simulink library "lib_ares"  (R2020a)
settings: Solver=VariableStepAuto  StartTime=0.0  StopTime=10.0  RelTol=1e-3
undefined symbols (not defined in the file or in its folder): DiscIntNeverNeededParam
libraries: simulink x9, $bdroot x6
(part 2 of 2)

== system lib_ares/baro_alt_to_Ps ==
  note: Static Pressure (atmospheres) as a function of Baro Alt (ft)
      | (valid for Alt < 36089)
      | this is /delta
  baro_alt_ft : Inport
  baro_alt_ft_to_Ps_atm : Fcn  Expr=(1.0-(u*(0.00356616/518.67)))^5.2561
  Ps_atm : Outport
  wires:
  baro_alt_ft/1 -> baro_alt_ft_to_Ps_atm/1
  baro_alt_ft_to_Ps_atm/1 -> Ps_atm/1

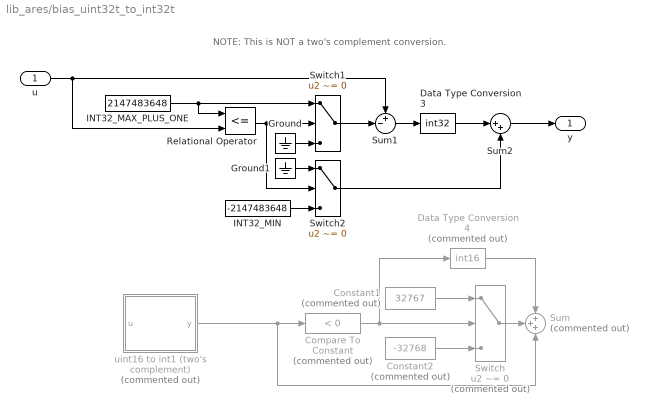
== system lib_ares/bias_uint32t_to_int32t ==
  note: NOTE: This is NOT a two's complement conversion.
  u : Inport  OutDataTypeStr=uint32
  Compare To Constant : simulink/Logic and Bit Operations/Compare To Constant  Commented=on  relop=<  const=0  OutDataTypeStr=boolean
  Constant1 : Constant  Commented=on  Value=32767  VectorParams1D=off  OutDataTypeStr=int16  SampleTime=1e-6
  Constant2 : Constant  Commented=on  Value=-32768  OutDataTypeStr=int16  SampleTime=1e-6
  Data Type Conversion3 : DataTypeConversion  OutDataTypeStr=int32  SaturateOnIntegerOverflow=on
  Data Type Conversion4 : DataTypeConversion  Commented=on  OutDataTypeStr=int16  SaturateOnIntegerOverflow=on
  Ground : Ground
  Ground1 : Ground
  INT32_MAX_PLUS_ONE : Constant  Value=2147483648  OutDataTypeStr=uint32
  INT32_MIN : Constant  Value=-2147483648  OutDataTypeStr=int32
  Relational Operator : RelationalOperator  Operator=<=  OutDataTypeStr=boolean  RndMeth=Simplest
  Sum : Sum  Commented=on  Inputs=+++
  Sum1 : Sum  Inputs=+-|
  Sum2 : Sum  Inputs=|++
  Switch : Switch  Commented=on  Criteria=u2 ~= 0
  Switch1 : Switch  Criteria=u2 ~= 0
  Switch2 : Switch  Criteria=u2 ~= 0
  uint16 to int1 (two's complement) : Subsystem  Commented=on
  y : Outport  OutDataTypeStr=int32
  wires:
  uint16 to int1 (two's complement)/1(y) -> Compare To Constant/1, Sum/3
  Data Type Conversion4/1 -> Sum/1
  Compare To Constant/1 -> Switch/2, Data Type Conversion4/1
  Constant2/1 -> Switch/3
  Constant1/1 -> Switch/1
  Switch/1 -> Sum/2
  ? -> uint16 to int1 (two's complement)/1(u)
  Sum2/1 -> y/1
  Switch1/1 -> Sum1/2
  INT32_MIN/1 -> Switch2/3
  INT32_MAX_PLUS_ONE/1 -> Relational Operator/1, Switch1/1
  Sum1/1 -> Data Type Conversion3/1
  Relational Operator/1 -> Switch1/2, Switch2/2
  Data Type Conversion3/1 -> Sum2/1
  Switch2/1 -> Sum2/2
  Ground/1 -> Switch1/3
  Ground1/1 -> Switch2/1
  u/1 -> Sum1/1, Relational Operator/2

== system lib_ares/cas_to_mach ==
  note: Mach number as a function of
      | calibrated airspeed (ft/s)
      |
      | NASA Reference Publication 1046, Pg.15 Speed of Sound
  cas_fps : Inport
  Divide : Product  Inputs=*/
  "Speed of Sound, fps, Sea Level Standard" : Constant  Value=1116.450  OutDataTypeStr=Inherit: Inherit via back propagation
  mach : Outport
  wires:
  "Speed of Sound, fps, Sea Level Standard"/1 -> Divide/2
  cas_fps/1 -> Divide/1
  Divide/1 -> mach/1

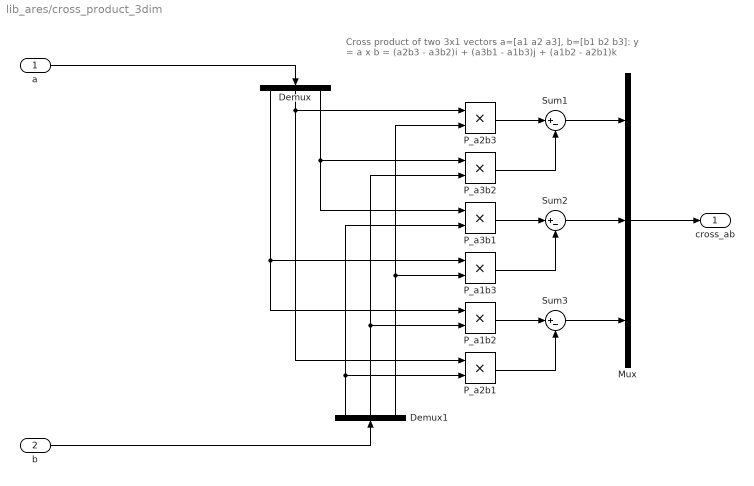
== system lib_ares/cross_product_3dim ==
  note: Cross product of two 3x1 vectors a=[a1 a2 a3], b=[b1 b2 b3]:
      | y = a x b = (a2b3 - a3b2)i + (a3b1 - a1b3)j + (a1b2 - a2b1)k
  a : Inport
  b : Inport  Port=2
  Demux : Demux  Outputs=3
  Demux1 : Demux  Outputs=3
  Mux : Mux  Inputs=3
  P_a1b2 : Product
  P_a1b3 : Product
  P_a2b1 : Product
  P_a2b3 : Product
  P_a3b1 : Product
  P_a3b2 : Product
  Sum1 : Sum  Inputs=|+-
  Sum2 : Sum  Inputs=|+-
  Sum3 : Sum  Inputs=|+-
  cross_ab : Outport
  wires:
  Demux/1 -> P_a1b3/1, P_a1b2/1
  Demux1/1 -> P_a3b1/2, P_a2b1/2
  Demux/2 -> P_a2b1/1, P_a2b3/1
  Demux/3 -> P_a3b1/1, P_a3b2/1
  P_a1b3/1 -> Sum2/2
  P_a2b1/1 -> Sum3/2
  P_a1b2/1 -> Sum3/1
  Demux1/3 -> P_a2b3/2, P_a1b3/2
  Demux1/2 -> P_a3b2/2, P_a1b2/2
  P_a3b2/1 -> Sum1/2
  P_a3b1/1 -> Sum2/1
  P_a2b3/1 -> Sum1/1
  Sum2/1 -> Mux/2
  Sum1/1 -> Mux/1
  Sum3/1 -> Mux/3
  b/1 -> Demux1/1
  a/1 -> Demux/1
  Mux/1 -> cross_ab/1

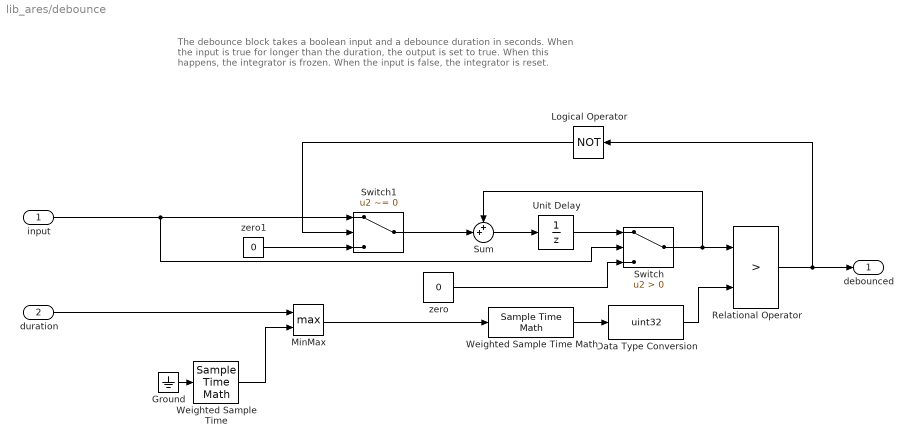
== system lib_ares/debounce ==
  note: The debounce block takes a boolean input and a debounce duration in seconds.
      |
      | When the input is true for longer than the duration, the output is set to true. When
      | this happens, the integrator is frozen. When the input is false, the integrator is
      | reset.
  input : Inport  OutDataTypeStr=boolean
  duration : Inport  Port=2
  Data Type Conversion : DataTypeConversion  OutDataTypeStr=uint32
  Ground : Ground
  Logical Operator : Logic  Operator=NOT  AllPortsSameDT=off  OutDataTypeStr=boolean
  MinMax : MinMax  Function=max  Inputs=2
  Relational Operator : RelationalOperator  Operator=>  OutDataTypeStr=boolean  RndMeth=Simplest
  Sum : Sum  Inputs=++|
  Switch : Switch  Criteria=u2 > Threshold
  Switch1 : Switch  Criteria=u2 ~= 0
  Unit Delay : UnitDelay  SampleTime=-1  HasFrameUpgradeWarning=on
  Weighted Sample Time : SampleTimeMath  TsampMathOp=Ts Only
  Weighted Sample Time Math : SampleTimeMath  TsampMathOp=/
  zero : Constant  Value=0  OutDataTypeStr=uint32
  zero1 : Constant  Value=0  OutDataTypeStr=uint32
  debounced : Outport  VectorParamsAs1DForOutWhenUnconnected=off
  wires:
  zero1/1 -> Switch1/3
  Logical Operator/1 -> Switch1/2
  Switch1/1 -> Sum/2
  input/1 -> Switch1/1, Switch/2
  Switch/1 -> Relational Operator/1, Sum/1
  Unit Delay/1 -> Switch/1
  Weighted Sample Time Math/1 -> Data Type Conversion/1
  zero/1 -> Switch/3
  Sum/1 -> Unit Delay/1
  duration/1 -> MinMax/1
  Relational Operator/1 -> debounced/1, Logical Operator/1
  MinMax/1 -> Weighted Sample Time Math/1
  Weighted Sample Time/1 -> MinMax/2
  Ground/1 -> Weighted Sample Time/1
  Data Type Conversion/1 -> Relational Operator/2

== system lib_ares/fta_handler_non_persistent ==
  input : Inport
  id : Inport  Port=2
  enable : Inport  Port=3
  Data Type Duplicate : DataTypeDuplicate
  Logical Operator3 : Logic  AllPortsSameDT=off  OutDataTypeStr=boolean
  Relational Operator2 : RelationalOperator  Operator===  OutDataTypeStr=boolean  RndMeth=Simplest
  Switch3 : Switch  Criteria=u2 ~= 0
  default_value_IC : Constant  Value=default_value  OutDataTypeStr=Inherit: Inherit via back propagation
  id_int32 : Constant  Value=id  OutDataTypeStr=int32
  output : Outport
  wires:
  id_int32/1 -> Relational Operator2/1
  input/1 -> Data Type Duplicate/1, Switch3/1  "new_value"
  Relational Operator2/1 -> Logical Operator3/1
  Switch3/1 -> output/1
  id/1 -> Relational Operator2/2
  enable/1 -> Logical Operator3/2
  default_value_IC/1 -> Data Type Duplicate/2, Switch3/3  "default_value"
  Logical Operator3/1 -> Switch3/2

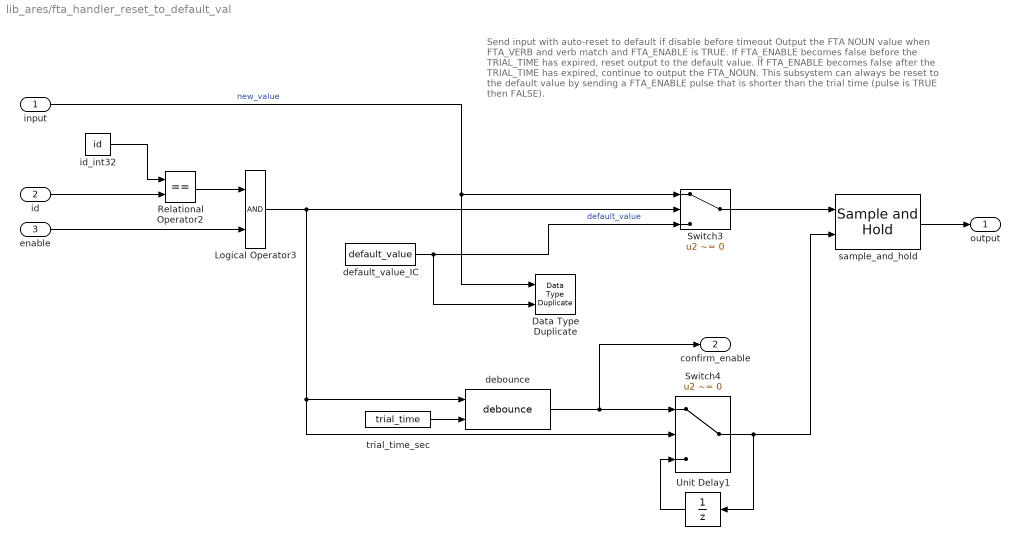
== system lib_ares/fta_handler_reset_to_default_val ==
  note: Send input with auto-reset to default if disable before timeout
      |
      | Output the FTA NOUN value when FTA_VERB and verb match and FTA_ENABLE is TRUE.
      | If FTA_ENABLE becomes false before the TRIAL_TIME has expired, reset output to the
      | default value. If FTA_ENABLE becomes false after the TRIAL_TIME has expired, continue
      | to output the FTA_NOUN.
      |
      | This subsystem can always be reset to the default value by sending a FTA_ENABLE pulse
      | that is shorter than the trial time (pulse is TRUE then FALSE).
  input : Inport
  id : Inport  Port=2
  enable : Inport  Port=3
  Data Type Duplicate : DataTypeDuplicate
  Logical Operator3 : Logic  AllPortsSameDT=off  OutDataTypeStr=boolean
  Relational Operator2 : RelationalOperator  Operator===  OutDataTypeStr=boolean  RndMeth=Simplest
  Switch3 : Switch  Criteria=u2 ~= 0
  Switch4 : Switch  Criteria=u2 ~= 0
  Unit Delay1 : UnitDelay  SampleTime=-1  HasFrameUpgradeWarning=on
  debounce : $bdroot/debounce  SystemSampleTime=-1  Latency=0  AutoFrameSizeCalculation=off
  default_value_IC : Constant  Value=default_value  OutDataTypeStr=Inherit: Inherit via back propagation
  id_int32 : Constant  Value=id  OutDataTypeStr=int32
  sample_and_hold : $bdroot/Sample and Hold  SystemSampleTime=-1  Latency=0  AutoFrameSizeCalculation=off
  trial_time_sec : Constant  Value=trial_time  OutDataTypeStr=Inherit: Inherit via back propagation
  output : Outport
  confirm_enable : Outport  Port=2
  wires:
  Logical Operator3/1 -> debounce/1, Switch4/2, Switch3/2
  debounce/1 -> confirm_enable/1, Switch4/1
  Unit Delay1/1 -> Switch4/3
  default_value_IC/1 -> Data Type Duplicate/2, Switch3/3  "default_value"
  enable/1 -> Logical Operator3/2
  id/1 -> Relational Operator2/2
  sample_and_hold/1 -> output/1
  Relational Operator2/1 -> Logical Operator3/1
  trial_time_sec/1 -> debounce/2
  Switch3/1 -> sample_and_hold/1
  input/1 -> Data Type Duplicate/1, Switch3/1  "new_value"
  id_int32/1 -> Relational Operator2/1
  Switch4/1 -> sample_and_hold/2, Unit Delay1/1

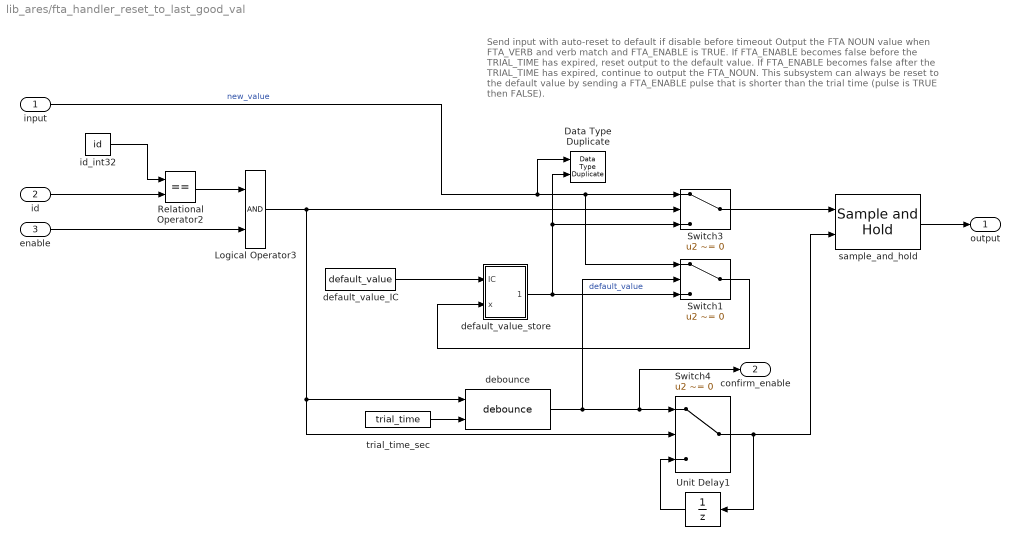
== system lib_ares/fta_handler_reset_to_last_good_val ==
  note: Send input with auto-reset to default if disable before timeout
      |
      | Output the FTA NOUN value when FTA_VERB and verb match and FTA_ENABLE is TRUE.
      | If FTA_ENABLE becomes false before the TRIAL_TIME has expired, reset output to the
      | default value. If FTA_ENABLE becomes false after the TRIAL_TIME has expired, continue
      | to output the FTA_NOUN.
      |
      | This subsystem can always be reset to the default value by sending a FTA_ENABLE pulse
      | that is shorter than the trial time (pulse is TRUE then FALSE).
  input : Inport
  id : Inport  Port=2
  enable : Inport  Port=3
  Data Type Duplicate : DataTypeDuplicate
  Logical Operator3 : Logic  AllPortsSameDT=off  OutDataTypeStr=boolean
  Relational Operator2 : RelationalOperator  Operator===  OutDataTypeStr=boolean  RndMeth=Simplest
  Switch1 : Switch  Criteria=u2 ~= 0
  Switch3 : Switch  Criteria=u2 ~= 0
  Switch4 : Switch  Criteria=u2 ~= 0
  Unit Delay1 : UnitDelay  SampleTime=-1  HasFrameUpgradeWarning=on
  debounce : $bdroot/debounce  SystemSampleTime=-1  Latency=0  AutoFrameSizeCalculation=off
  default_value_IC : Constant  Value=default_value  OutDataTypeStr=Inherit: Inherit via back propagation
  default_value_store : Subsystem
  id_int32 : Constant  Value=id  OutDataTypeStr=int32
  sample_and_hold : $bdroot/Sample and Hold  SystemSampleTime=-1  Latency=0  AutoFrameSizeCalculation=off
  trial_time_sec : Constant  Value=trial_time  OutDataTypeStr=Inherit: Inherit via back propagation
  output : Outport
  confirm_enable : Outport  Port=2
  wires:
  default_value_IC/1 -> default_value_store/1(IC)
  Switch4/1 -> Unit Delay1/1, sample_and_hold/2
  id_int32/1 -> Relational Operator2/1
  input/1 -> Switch3/1, Switch1/1, Data Type Duplicate/1  "new_value"
  Switch3/1 -> sample_and_hold/1
  trial_time_sec/1 -> debounce/2
  Relational Operator2/1 -> Logical Operator3/1
  sample_and_hold/1 -> output/1
  id/1 -> Relational Operator2/2
  enable/1 -> Logical Operator3/2
  default_value_store/1(Out1) -> Switch1/3, Data Type Duplicate/2, Switch3/3  "default_value"
  Switch1/1 -> default_value_store/2(x)
  Unit Delay1/1 -> Switch4/3
  debounce/1 -> confirm_enable/1, Switch4/1, Switch1/2
  Logical Operator3/1 -> Switch3/2, Switch4/2, debounce/1

== system lib_ares/mach_oat_to_tas ==
  note: True airspeed (ft/s) as a function of mach and outside air temp (R)
  mach : Inport
  oat_R : Inport  Port=2
  Divide : Product  Inputs=*/
  Product : Product  Inputs=3
  Sqrt : Sqrt  SaturateOnIntegerOverflow=on
  Tstd_rankine : Constant  Value=518.67  OutDataTypeStr=Inherit: Inherit via back propagation
  speed_of_sound_fps : Constant  Value=1116.450  OutDataTypeStr=Inherit: Inherit via back propagation
  tas_fps : Outport
  wires:
  mach/1 -> Product/1
  Tstd_rankine/1 -> Divide/2
  oat_R/1 -> Divide/1
  Divide/1 -> Sqrt/1
  Product/1 -> tas_fps/1
  Sqrt/1 -> Product/3
  speed_of_sound_fps/1 -> Product/2

== system lib_ares/mach_to_Qc ==
  note: Impact Pressure (Qc) (atmospheres) as a
      | function of mach number
      | (valid for mach < 1)
      |
      | NASA Reference Publication 1046, Eq. 3.25
  mach : Inport
  mach_to_Qc_atm : Fcn  Expr=(1.0 + 0.2*u^2 )^(7/2) - 1.0
  Qc_atm : Outport
  wires:
  mach/1 -> mach_to_Qc_atm/1
  mach_to_Qc_atm/1 -> Qc_atm/1

== system lib_ares/mach_to_cas ==
  note: Calibrated airspeed (ft/s) as a function of
      | Mach number
      |
      | NASA Reference Publication 1046, Pg.15 Speed of Sound
  mach : Inport
  Product : Product
  "Speed of Sound, fps, Sea Level Standard" : Constant  Value=1116.450  OutDataTypeStr=Inherit: Inherit via back propagation
  cas_fps : Outport
  wires:
  Product/1 -> cas_fps/1
  "Speed of Sound, fps, Sea Level Standard"/1 -> Product/2
  mach/1 -> Product/1

== system lib_ares/mean ==
  In1 : Inport
  In2 : Inport  Port=2
  Add : Sum
  Gain2 : Gain  Gain=0.5
  mean : Outport
  wires:
  Gain2/1 -> mean/1
  In2/1 -> Add/2
  In1/1 -> Add/1
  Add/1 -> Gain2/1

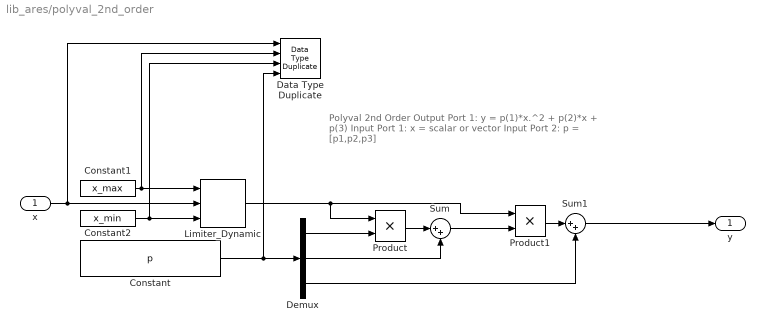
== system lib_ares/polyval_2nd_order ==
  note: Polyval 2nd Order
      |
      | Output Port 1: y = p(1)*x.^2 + p(2)*x + p(3)
      |
      | Input Port 1: x = scalar or vector
      | Input Port 2: p = [p1,p2,p3]
  x : Inport
  Constant : Constant  Value=p  OutDataTypeStr=Inherit: Inherit via back propagation
  Constant1 : Constant  Value=x_max  OutDataTypeStr=Inherit: Inherit via back propagation
  Constant2 : Constant  Value=x_min  OutDataTypeStr=Inherit: Inherit via back propagation
  Data Type Duplicate : DataTypeDuplicate  DisableCoverage=on  NumInputPorts=4
  Demux : Demux  Outputs=3
  Limiter_Dynamic : $bdroot/Limiter_Dynamic
  Product : Product
  Product1 : Product
  Sum : Sum  Inputs=|++
  Sum1 : Sum  Inputs=|++
  y : Outport
  wires:
  Sum1/1 -> y/1
  Demux/1 -> Product/2
  Constant/1 -> Data Type Duplicate/4, Demux/1
  Product1/1 -> Sum1/1
  Demux/2 -> Sum/2
  Demux/3 -> Sum1/2
  Limiter_Dynamic/1 -> Product/1, Product1/1
  Product/1 -> Sum/1
  Sum/1 -> Product1/2
  x/1 -> Data Type Duplicate/1, Limiter_Dynamic/2
  Constant1/1 -> Data Type Duplicate/2, Limiter_Dynamic/1
  Constant2/1 -> Data Type Duplicate/3, Limiter_Dynamic/3

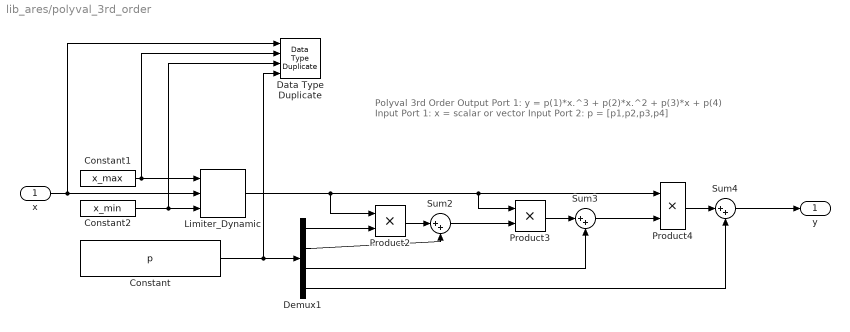
== system lib_ares/polyval_3rd_order ==
  note: Polyval 3rd Order
      |
      | Output Port 1: y = p(1)*x.^3 + p(2)*x.^2 + p(3)*x + p(4)
      |
      | Input Port 1: x = scalar or vector
      | Input Port 2: p = [p1,p2,p3,p4]
  x : Inport
  Constant : Constant  Value=p  OutDataTypeStr=Inherit: Inherit via back propagation
  Constant1 : Constant  Value=x_max  OutDataTypeStr=Inherit: Inherit via back propagation
  Constant2 : Constant  Value=x_min  OutDataTypeStr=Inherit: Inherit via back propagation
  Data Type Duplicate : DataTypeDuplicate  DisableCoverage=on  NumInputPorts=4
  Demux1 : Demux
  Limiter_Dynamic : $bdroot/Limiter_Dynamic
  Product2 : Product
  Product3 : Product
  Product4 : Product
  Sum2 : Sum  Inputs=|++
  Sum3 : Sum  Inputs=|++
  Sum4 : Sum  Inputs=|++
  y : Outport
  wires:
  Constant/1 -> Demux1/1, Data Type Duplicate/4
  x/1 -> Data Type Duplicate/1, Limiter_Dynamic/2
  Constant1/1 -> Data Type Duplicate/2, Limiter_Dynamic/1
  Constant2/1 -> Data Type Duplicate/3, Limiter_Dynamic/3
  Demux1/1 -> Product2/2
  Demux1/2 -> Sum2/2
  Sum3/1 -> Product4/2
  Product2/1 -> Sum2/1
  Sum2/1 -> Product3/2
  Limiter_Dynamic/1 -> Product4/1, Product3/1, Product2/1
  Product4/1 -> Sum4/1
  Product3/1 -> Sum3/1
  Demux1/3 -> Sum3/2
  Sum4/1 -> y/1
  Demux1/4 -> Sum4/2

== system lib_ares/select_middle_value ==
  A : Inport
  B : Inport  Port=2
  C : Inport  Port=3
  MinMax1 : MinMax  Inputs=2
  MinMax2 : MinMax  Function=max  Inputs=2
  MinMax3 : MinMax  Inputs=2
  MinMax4 : MinMax  Inputs=2
  MinMax5 : MinMax  Function=max  Inputs=2
  mid_value : Outport
  wires:
  A/1 -> MinMax4/1, MinMax1/1
  B/1 -> MinMax3/1, MinMax4/2
  C/1 -> MinMax1/2, MinMax3/2
  MinMax1/1 -> MinMax5/1
  MinMax3/1 -> MinMax2/1
  MinMax4/1 -> MinMax2/2
  MinMax2/1 -> MinMax5/2
  MinMax5/1 -> mid_value/1

== system lib_ares/table_lookup_1d ==
  In1 : Inport
  1-D Lookup Table : Lookup_n-D  NumberOfTableDimensions=1  BreakpointsForDimension1=xdat  BeginIndexSearchUsingPreviousIndexResult=on  Table=ydat  ExtrapMethod=Clip  UseLastTableValue=on  InternalRulePriority=Speed  RndMeth=Simplest  InputSameDT=on
  Out1 : Outport
  wires:
  In1/1 -> 1-D Lookup Table/1
  1-D Lookup Table/1 -> Out1/1

== system lib_ares/tas_oat_to_mach ==
  note: Mach as a function of True airspeed (ft/s) and outside air temp (R)
  tas_fps : Inport
  oat_R : Inport  Port=2
  Divide : Product  Inputs=*/
  Divide1 : Product  Inputs=*/
  Product : Product
  Sqrt : Sqrt  SaturateOnIntegerOverflow=on
  Tstd_rankine : Constant  Value=518.67  OutDataTypeStr=Inherit: Inherit via back propagation
  speed_of_sound_fps : Constant  Value=1116.450  OutDataTypeStr=Inherit: Inherit via back propagation
  mach : Outport
  wires:
  Divide1/1 -> mach/1
  tas_fps/1 -> Divide1/1
  Tstd_rankine/1 -> Divide/2
  oat_R/1 -> Divide/1
  Product/1 -> Divide1/2
  Sqrt/1 -> Product/2
  speed_of_sound_fps/1 -> Product/1
  Divide/1 -> Sqrt/1

== system lib_ares/bias_uint32t_to_int32t/uint16 to int1 (two's complement) ==
  u : Inport
  Bit Clear : simulink/Logic and Bit Operations/Bit Clear  iBit=15
      settings: SourceProductBaseCode=SL
  Constant2 : Constant  Value=-2^15  OutDataTypeStr=int16  SampleTime=1e-6
  Data Type Conversion1 : DataTypeConversion  OutDataTypeStr=int16
  Extract Bits : simulink/Logic and Bit Operations/Extract Bits  bitsToExtract=Range of bits  numBits=8  bitIdxRange=15  outScalingMode=Treat bit field as an integer
  Product : Product  RndMeth=Zero
  Sum : Sum  Inputs=|++
  y : Outport
  wires:
  u/1 -> Extract Bits/1, Bit Clear/1
  Product/1 -> Sum/2
  Extract Bits/1 -> Product/2
  Constant2/1 -> Product/1
  Sum/1 -> y/1
  Data Type Conversion1/1 -> Sum/1
  Bit Clear/1 -> Data Type Conversion1/1

== system lib_ares/fta_handler_reset_to_last_good_val/default_value_store ==
  IC : Inport
  x : Inport  Port=2
  Constant : Constant  Value=0  OutDataTypeStr=Inherit: Inherit via back propagation
  Switch1 : Switch  Criteria=u2 ~= 0
  Unit Delay1 : UnitDelay  SampleTime=-1  HasFrameUpgradeWarning=on
  initialize_store : UnitDelay  InitialCondition=1  SampleTime=-1  HasFrameUpgradeWarning=on
  Out1 : Outport
  wires:
  Unit Delay1/1 -> Switch1/3
  x/1 -> Unit Delay1/1
  IC/1 -> Switch1/1
  Switch1/1 -> Out1/1
  Constant/1 -> initialize_store/1
  initialize_store/1 -> Switch1/2
